simulink model "sf_matrix"  (Simulink 7.6)
settings: Solver=ode45  StartTime=0.0  StopTime=1  MaxStep=1  RelTol=1e-3
settings Model: Creator=The MathWorks Inc.  CovMetricSettings=dcmtr  ExtModeAutoUpdateStatusClock=off
settings OptimizationCC: BooleanDataType=off  InlineInvariantSignals=on  InitFltsAndDblsToZero=on  EfficientMapNaN2IntZero=off
settings DebuggingCC: SaveWithParameterizedLinksMsg=none  SignalResolutionControl=TryResolveAllWithWarning  SolverPrmCheckMsg=none  MultiTaskDSMMsg=warning  MultiTaskCondExecSysMsg=none  StrictBusMsg=None
settings HardwareCC: TargetUnknown=on
settings SFSimCC: SimParseCustomCode=off
settings RTWCC: IncludeERTFirstTime=on
settings GRTTargetCC: TargetFcnLib=ansi_tfl_tmw.mat

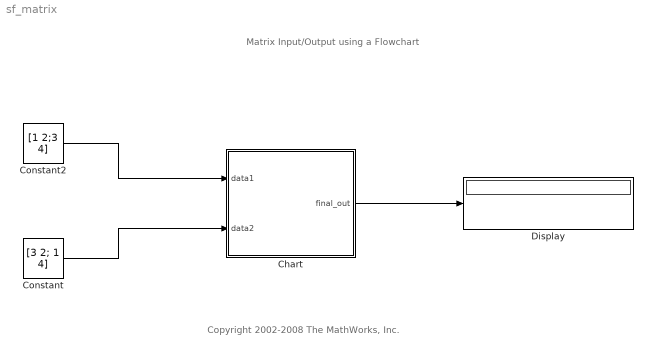
== system sf_matrix ==
  note: Matrix Input/Output using a Flowchart
  note: Copyright 2002-2008 The MathWorks, Inc.
  Chart : Stateflow chart  TreatAsAtomicUnit=on
  Constant : Constant  Value=[3 2; 1 4]  VectorParams1D=off
  Constant2 : Constant  Value=[1 2;3 4]  VectorParams1D=off
  Display : Display
  wires:
  Constant2/1 -> Chart/1(data1)
  Constant/1 -> Chart/2(data2)
  Chart/1(final_out) -> Display/1

== stateflow chart Chart ==
  note: Equivalent C-Code:
      |
      | for(i=0;i<2;i++)
      |    for(j=0;j<2;j++)
      |        {
      |          int final_out[2][2];
      |          final_out[i][j]=(data1[i][0]*data2[0][j])+(data1[i][1]+data2[1][j]);
      |        }
  (default) -> (junction 4) : {final_out[0][0]=(data1[0][0]*data2[0][0])+(data1[0][1]*data2[1][0]);}
  (junction 4) -> (junction 5) : {final_out[0][1]=(data1[0][0]*data2[0][1])+(data1[0][1]*data2[1][1]);}
  (junction 5) -> (junction 6) : {final_out[1][0]=(data1[1][0]*data2[0][0])+(data1[1][1]*data2[1][0]);}
  (junction 6) -> (junction 7) : {final_out[1][1]=(data1[1][0]*data2[0][1])+(data1[1][1]*data2[1][1]);}
  (junction 7) -> (junction 8)
  data: final_out output double size=[2 2]; data1 input double size=[2 2]; data2 input double size=[2 2]
